simulink model "controlporvelocidad"  (R2023a)
settings: Solver=VariableStepAuto  StartTime=0.0  StopTime=10.0  RelTol=1e-3
settings Model: Creator=Jimmy  LastModifiedBy=Jimmy

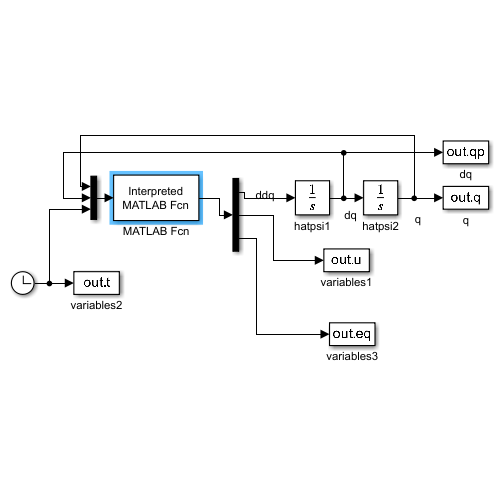
[thumbnail: Simulink's stored preview of the top-level diagram]
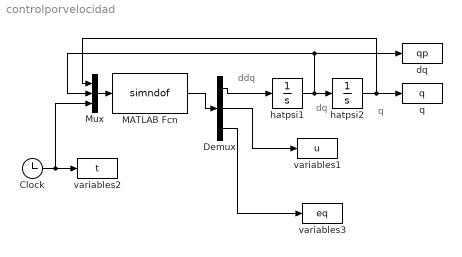
== system controlporvelocidad ==
  note: dq
  note: ddq
  note: q
  Clock : Clock
  Demux : Demux  Outputs=[2;2;2]
  MATLAB Fcn : MATLABFcn  MATLABFcn=simndof  OutputDimensions=6
  Mux : Mux  Inputs=3
  dq : ToWorkspace  VariableName=qp  SampleTime=-1
  hatpsi1 : Integrator  InitialCondition=[0;0]
  hatpsi2 : Integrator  InitialCondition=[-pi/8;pi/2]
  q : ToWorkspace  VariableName=q  SampleTime=-1
  variables1 : ToWorkspace  VariableName=u  SampleTime=-1
  variables2 : ToWorkspace  VariableName=t  SampleTime=-1
  variables3 : ToWorkspace  VariableName=eq  SampleTime=-1
  wires:
  MATLAB Fcn/1 -> Demux/1
  Demux/2 -> variables1/1
  Demux/3 -> variables3/1
  hatpsi2/1 -> Mux/1, q/1
  hatpsi1/1 -> Mux/2, dq/1, hatpsi2/1
  Mux/1 -> MATLAB Fcn/1
  Demux/1 -> hatpsi1/1
  Clock/1 -> Mux/3, variables2/1
